simulink model "ee463_project_simulationV4"  (R2023b)
settings: Solver=VariableStepAuto  StartTime=0.0  StopTime=0.04  RelTol=1e-3
undefined symbols (not defined in the file or in its folder): Acid, Lead
libraries: spsDiodeLib x8, spsVoltageMeasurementLib x7, spsMeanLib x6, spsCurrentMeasurementLib x5, spsSeriesRLCBranchLib x5, spsACVoltageSourceLib x3, spsBatteryLib x1, spsMosfetLib x1, spsRMSLib x1, sps_lib x1
settings Model: Creator=Emir  LastModifiedBy=Emir

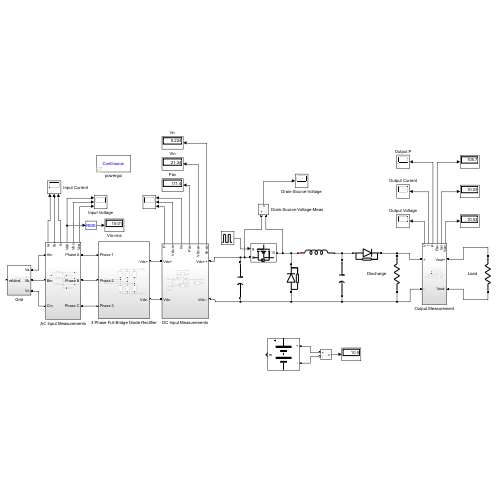
[thumbnail: Simulink's stored preview of the top-level diagram]
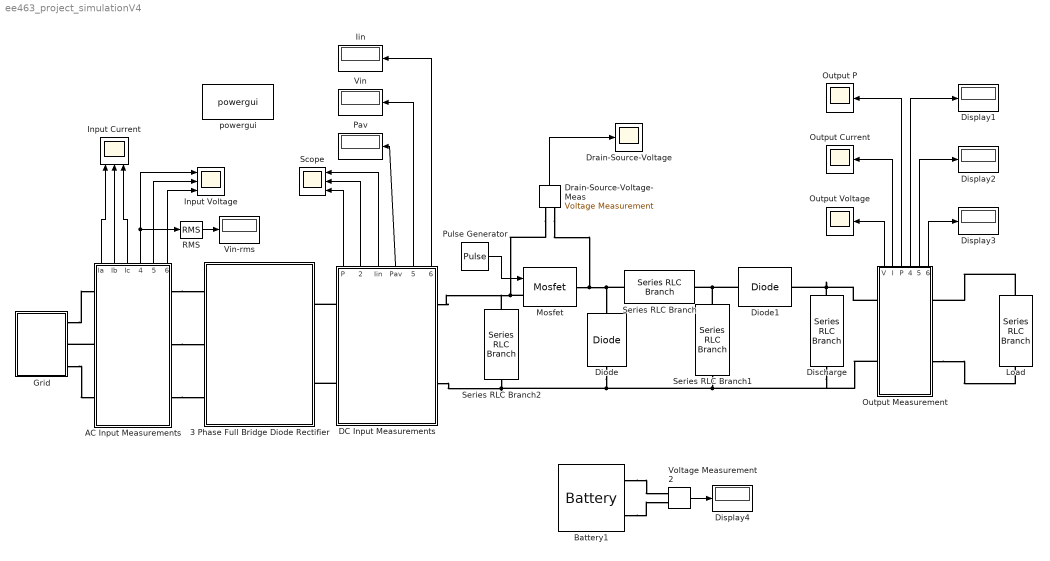
== system ee463_project_simulationV4 ==
  3 Phase Full Bridge Diode Rectifier : Subsystem
  AC Input Measurements : Subsystem
      settings: PortSchema="{\"entries\":[{\"content\":{\"sides\":[{\"content\":{\"connectorIds\":[\"LConn1\",\"LConn2\",\"LConn3\"]},\"type\":\"ConnectorPlacement.EquallySpacedRectSide\",\"uuid\":\"04a5a0c8-76ab-4056-bfdd-b703a3d2aa28\"},{\"content\":{\"connectorIds\":[\"RConn1\",\"RConn2\",\"RConn3\"],\"side\":\"RIGHT\"},\"type\":\"ConnectorPlacement.EquallySpacedRectSide\",\"uuid\":\"3565172a-00f9-43c9-81c3-3e47c8c41d3a\"},{\"content\":{\"connectorIds\":[\"Out1\",\"Out2\",\"Out3\",\"Out4\",\"Out5\",\"Out6\"],\"side\":\"TOP\"},\"type\":\"ConnectorPlacement.EquallySpacedRectSide\",\"uuid\":\"dbadec88-7628-4dba-94e1-272ca81af1aa\"},{\"content\":{\"side\":\"BOTTOM\"},\"type\":\"ConnectorPlacement.EquallySpacedRectSide\",\"uuid\":\"5d01f6b5-6790-4bc6-9328-17bbb75a6f10\"}]},\"type\":\"ConnectorPlacement.EquallySpacedConnector\",\"uuid\":\"addb2cae-2f57-4e8c-a556-dd1f5358b3e0\"}],\"packageUris\":[\"http://schema.mathworks.com/mf0/Connector/R2020b\"],\"version\":\"1.0\"}"
  Battery1 : spsBatteryLib/Battery  BatType=Lead-Acid  ShowTempParam=off  ThermalPreset=no  ShowAgeParam=off  NomV=12  NomQ=100  SOC=10  Batt_Tr=30  PresetModel=on  MaxQ=104.1667  MinV=9  FullV=13.0658  Dis_rate=20  R=0.0012  Normal_OP=31.0278  expZone="[12.2171     0.333333]"  current=[6.5 13 32.5]  Units=Time  Tci=20  NomT=20  T2=-30  MaxQ2=4.8  FullV2=7.1  Normal_OP2=5.655  expZone2="[6.58           1]"  Rca=0.6  ti=2000  Dp=0  Neq0=0  Tsim=1e6  Ta1=25  Qeol=5.4*0.9  Reol=0.013333*1.2  Char_age=[2.3478, 3]  Dis_age=[2.3478, 10]  N1=1500  N2=10500  N3=1000  N4=1400  Ta2=45  N5=950
  DC Input Measurements : Subsystem
      settings: PortSchema="{\"entries\":[{\"content\":{\"sides\":[{\"content\":{\"connectorIds\":[\"LConn1\",\"LConn2\"]},\"type\":\"ConnectorPlacement.EquallySpacedRectSide\",\"uuid\":\"d21f3327-f92a-42ff-962f-d2a0482b5819\"},{\"content\":{\"connectorIds\":[\"RConn1\",\"RConn2\"],\"side\":\"RIGHT\"},\"type\":\"ConnectorPlacement.EquallySpacedRectSide\",\"uuid\":\"4cc980a8-4b33-4409-8260-8c3cf4970e9e\"},{\"content\":{\"connectorIds\":[\"Out1\",\"Out2\",\"Out3\",\"Out4\",\"Out5\",\"Out6\"],\"side\":\"TOP\"},\"type\":\"ConnectorPlacement.EquallySpacedRectSide\",\"uuid\":\"010d1ec9-7ee7-4226-b983-8384f0725a58\"},{\"content\":{\"side\":\"BOTTOM\"},\"type\":\"ConnectorPlacement.EquallySpacedRectSide\",\"uuid\":\"5c959f18-9408-4ec5-8d60-b5cac5d211f5\"}]},\"type\":\"ConnectorPlacement.EquallySpacedConnector\",\"uuid\":\"5b7df6e5-50e0-402e-8feb-d27b87324437\"}],\"packageUris\":[\"http://schema.mathworks.com/mf0/Connector/R2020b\"],\"version\":\"1.0\"}"
  Diode : spsDiodeLib/Diode  Ron=0.001  Lon=0  Vf=0.8  IC=0  UseSnubber=0  Rs=500  Cs=250e-9  Measurements=off
  Diode1 : spsDiodeLib/Diode  Ron=0.001  Lon=0  Vf=0.8  IC=0  UseSnubber=0  Rs=500  Cs=250e-9  Measurements=off
  Discharge : spsSeriesRLCBranchLib/Series RLC Branch  LConnTagsString=__new0  RConnTagsString=__new0  BranchType=R  Resistance=100000  Inductance=1e-3  SetiL0=off  InitialCurrent=0  Capacitance=1000e-6  Setx0=off  InitialVoltage=0  Measurements=None
  Display{1..4} (4 alike) : Display
  Drain-Source-Voltage : Scope
  Drain-Source-Voltage-Meas : spsVoltageMeasurementLib/Voltage Measurement  PhasorSimulation=off  OutputType=Complex  PSBequivalent=0
  Grid : Subsystem
  Iin : Display
  Input Current : Scope  NumInputPorts=3
  Input Voltage : Scope  NumInputPorts=3
  Load : spsSeriesRLCBranchLib/Series RLC Branch  LConnTagsString=__new0  RConnTagsString=__new0  BranchType=R  Resistance=1.05  Inductance=1e-3  SetiL0=off  InitialCurrent=0  Capacitance=1000e-6  Setx0=off  InitialVoltage=0  Measurements=None
  Mosfet : spsMosfetLib/Mosfet  Ron=0.1  Lon=0  Rd=0.01  Vfd=0  IC=0  Rs=1e5  Cs=inf  Measurements=off
  Output Current : Scope
  Output Measurement : Subsystem
      settings: PortSchema="{\"entries\":[{\"content\":{\"sides\":[{\"content\":{\"connectorIds\":[\"LConn1\",\"LConn2\"]},\"type\":\"ConnectorPlacement.EquallySpacedRectSide\",\"uuid\":\"5134c9a7-91fc-4055-8b38-7fcc39efd9ae\"},{\"content\":{\"connectorIds\":[\"RConn1\",\"RConn2\"],\"side\":\"RIGHT\"},\"type\":\"ConnectorPlacement.EquallySpacedRectSide\",\"uuid\":\"a0adcaf9-cd58-4f8e-859e-0ced41501c8a\"},{\"content\":{\"connectorIds\":[\"Out1\",\"Out2\",\"Out3\",\"Out4\",\"Out5\",\"Out6\"],\"side\":\"TOP\"},\"type\":\"ConnectorPlacement.EquallySpacedRectSide\",\"uuid\":\"15bd731c-c78b-43c7-93d7-93e7c2271690\"}]},\"type\":\"ConnectorPlacement.EquallySpacedConnector\",\"uuid\":\"f842e8ba-c63a-4c27-b4ce-14ca0dc73f48\"}],\"packageUris\":[\"http://schema.mathworks.com/mf0/Connector/R2020b\"],\"version\":\"1.0\"}"
  Output P : Scope
  Output Voltage : Scope
  Pav : Display
  Pulse Generator : DiscretePulseGenerator  PulseType=Time based  Period=1e-5  PulseWidth=51.84
  RMS : spsRMSLib/RMS  TrueRMS=on  Freq=60  RMSInit=120  Ts=0
  Scope : Scope  NumInputPorts=3
  Series RLC Branch : spsSeriesRLCBranchLib/Series RLC Branch  LConnTagsString=__new0  RConnTagsString=__new0  BranchType=L  Resistance=1  Inductance=100e-6  SetiL0=off  InitialCurrent=0  Capacitance=1e-6  Setx0=off  InitialVoltage=0  Measurements=None
  Series RLC Branch1 : spsSeriesRLCBranchLib/Series RLC Branch  LConnTagsString=__new0  RConnTagsString=__new0  BranchType=C  Resistance=100  Inductance=1e-3  SetiL0=off  InitialCurrent=0  Capacitance=5.6e-6  Setx0=off  InitialVoltage=0  Measurements=None
  Series RLC Branch2 : spsSeriesRLCBranchLib/Series RLC Branch  LConnTagsString=__new0  RConnTagsString=__new0  BranchType=C  Resistance=100  Inductance=1e-3  SetiL0=off  InitialCurrent=0  Capacitance=4000e-6  Setx0=off  InitialVoltage=0  Measurements=None
  Vin : Display
  Vin-rms : Display
  Voltage Measurement2 : spsVoltageMeasurementLib/Voltage Measurement  PhasorSimulation=off  OutputType=Complex  PSBequivalent=0
  powergui : sps_lib/powergui  Priority=1  SimulationMode=Continuous  SampleTime=50e-6  frequency=60  Iterations=50  frequencyindice=0  Pbase=100e6  ErrMax=1e-4  UnitsV=kV  UnitsW=MW  buscounter=0  FunctionMessages=off  echomessages=off  EnableUseOfTLC=off  CurrentSourceSwitches=off  DisableSnubberDevices=off  DisableRonSwitches=off  DisableVfSwitches=on  DisplayEquations=off  AutomaticDiscreteSolvers=off  SolverType=Tustin/Backward Euler (TBE)  Interpol=off  ExternalGateDelay=off  methode=off  Ts=100  x0status=blocks  SPID=on  SwTol=0  HookPort=off  NonlinearTolerance=1e-4  nMaxIteration=100  ContinueOnMaxIteration=off  RestoreLinks=warning  ResistiveCurrentMeasurement=off  Frange=[0:2:500]  Ylog=off  Xlog=on  ShowGrid=off  save=off  variable=ZData  structure=0  ZoomFFT=off  StartTime=0.0  cycles=1  DisplayStyle=1  fundamental=60  FreqAxis=off  MaxFrequency=1000  frequencyindicesteady=1  RmsSteady=1  display=off
  wires:
  Pulse Generator/1 -> Mosfet/1
  Drain-Source-Voltage-Meas/1 -> Drain-Source-Voltage/1
  AC Input Measurements/1(Ia) -> Input Current/1
  AC Input Measurements/4(Vab) -> Input Voltage/1, RMS/1
  AC Input Measurements/2(Ib) -> Input Current/2
  AC Input Measurements/5(Vbc) -> Input Voltage/2
  AC Input Measurements/3(Ic) -> Input Current/3
  RMS/1 -> Vin-rms/1
  Voltage Measurement2/1 -> Display4/1
  DC Input Measurements/5(Vdc-av) -> Vin/1
  DC Input Measurements/6(Iin-av) -> Iin/1
  DC Input Measurements/1(P) -> Scope/3
  DC Input Measurements/4(Pav) -> Pav/1
  AC Input Measurements/6(Vca) -> Input Voltage/3
  DC Input Measurements/2(Vdc-in) -> Scope/2
  DC Input Measurements/3(Iin) -> Scope/1
  Output Measurement/2(I) -> Output Current/1
  Output Measurement/1(V) -> Output Voltage/1
  Output Measurement/3(P) -> Output P/1
  Output Measurement/6(V-av) -> Display3/1
  Output Measurement/5(Iav) -> Display2/1
  Output Measurement/4(Pav) -> Display1/1
  connections:
  DC Input Measurements/LConn2 -- 3 Phase Full Bridge Diode Rectifier/RConn2
  Drain-Source-Voltage-Meas/LConn1 -- DC Input Measurements/RConn1 -- Series RLC Branch2/LConn1 -- Mosfet/LConn1
  Mosfet/RConn1 -- Series RLC Branch/LConn1 -- Diode/RConn1 -- Drain-Source-Voltage-Meas/LConn2
  Series RLC Branch1/LConn1 -- Diode1/LConn1 -- Series RLC Branch/RConn1
  AC Input Measurements/RConn1 -- 3 Phase Full Bridge Diode Rectifier/LConn1
  Grid/RConn1 -- AC Input Measurements/LConn1
  AC Input Measurements/LConn2 -- Grid/RConn2
  AC Input Measurements/RConn2 -- 3 Phase Full Bridge Diode Rectifier/LConn2
  Grid/RConn3 -- AC Input Measurements/LConn3
  AC Input Measurements/RConn3 -- 3 Phase Full Bridge Diode Rectifier/LConn3
  Battery1/LConn1 -- Voltage Measurement2/LConn1
  Battery1/LConn2 -- Voltage Measurement2/LConn2
  DC Input Measurements/LConn1 -- 3 Phase Full Bridge Diode Rectifier/RConn1
  Series RLC Branch1/RConn1 -- Discharge/RConn1 -- Output Measurement/LConn2 -- DC Input Measurements/RConn2 -- Series RLC Branch2/RConn1 -- Diode/LConn1
  Output Measurement/LConn1 -- Diode1/RConn1 -- Discharge/LConn1
  Load/LConn1 -- Output Measurement/RConn1
  Output Measurement/RConn2 -- Load/RConn1

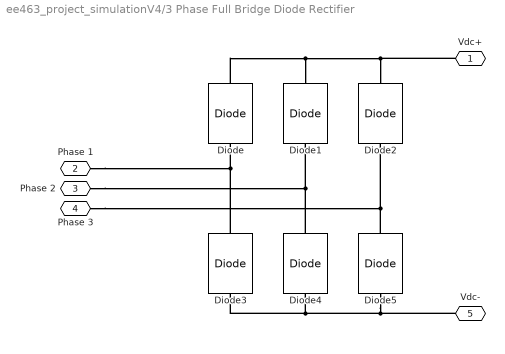
== system ee463_project_simulationV4/3 Phase Full Bridge Diode Rectifier ==
  Diode{,1..5} (6 alike) : spsDiodeLib/Diode  Ron=0.001  Lon=0  Vf=0.8  IC=0  UseSnubber=0  Rs=500  Cs=250e-9  Measurements=off
  Vdc+ : PMIOPort  Side=Right
  Phase 1 : PMIOPort  Port=2  Side=Left
  Phase 2 : PMIOPort  Port=3  Side=Left
  Phase 3 : PMIOPort  Port=4  Side=Left
  Vdc- : PMIOPort  Port=5  Side=Right
  connections:
  Diode4/RConn1 -- Phase 2/RConn1 -- Diode1/LConn1
  Diode5/RConn1 -- Phase 3/RConn1 -- Diode2/LConn1
  Diode/RConn1 -- Diode1/RConn1 -- Vdc+/RConn1 -- Diode2/RConn1
  Diode3/RConn1 -- Phase 1/RConn1 -- Diode/LConn1
  Diode5/LConn1 -- Vdc-/RConn1 -- Diode4/LConn1 -- Diode3/LConn1

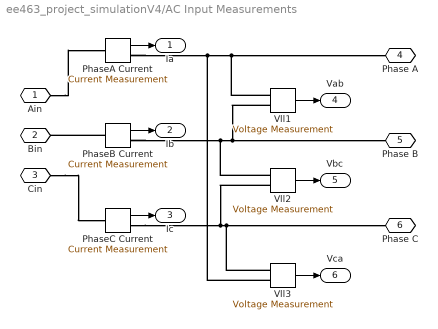
== system ee463_project_simulationV4/AC Input Measurements ==
  PhaseA Current : spsCurrentMeasurementLib/Current Measurement  PhasorSimulation=off  OutputType=Complex  PSBequivalent=0
  PhaseB Current : spsCurrentMeasurementLib/Current Measurement  PhasorSimulation=off  OutputType=Complex  PSBequivalent=0
  PhaseC Current : spsCurrentMeasurementLib/Current Measurement  PhasorSimulation=off  OutputType=Complex  PSBequivalent=0
  Vll1 : spsVoltageMeasurementLib/Voltage Measurement  PhasorSimulation=off  OutputType=Complex  PSBequivalent=0
  Vll2 : spsVoltageMeasurementLib/Voltage Measurement  PhasorSimulation=off  OutputType=Complex  PSBequivalent=0
  Vll3 : spsVoltageMeasurementLib/Voltage Measurement  PhasorSimulation=off  OutputType=Complex  PSBequivalent=0
  Ain : PMIOPort  Side=Left
  Bin : PMIOPort  Port=2  Side=Left
  Cin : PMIOPort  Port=3  Side=Left
  Phase A : PMIOPort  Port=4  Side=Right
  Phase B : PMIOPort  Port=5  Side=Right
  Phase C : PMIOPort  Port=6  Side=Right
  Ia : Outport
  Ib : Outport  Port=2
  Ic : Outport  Port=3
  Vab : Outport  Port=4
  Vbc : Outport  Port=5
  Vca : Outport  Port=6
  wires:
  PhaseC Current/1 -> Ic/1
  Vll3/1 -> Vca/1
  PhaseA Current/1 -> Ia/1
  PhaseB Current/1 -> Ib/1
  Vll1/1 -> Vab/1
  Vll2/1 -> Vbc/1
  connections:
  PhaseB Current/RConn1 -- Vll2/LConn1 -- Vll1/LConn2 -- Phase B/RConn1
  PhaseA Current/RConn1 -- Vll3/LConn2 -- Phase A/RConn1 -- Vll1/LConn1
  Cin/RConn1 -- PhaseC Current/LConn1
  Ain/RConn1 -- PhaseA Current/LConn1
  PhaseC Current/RConn1 -- Phase C/RConn1 -- Vll3/LConn1 -- Vll2/LConn2
  PhaseB Current/LConn1 -- Bin/RConn1

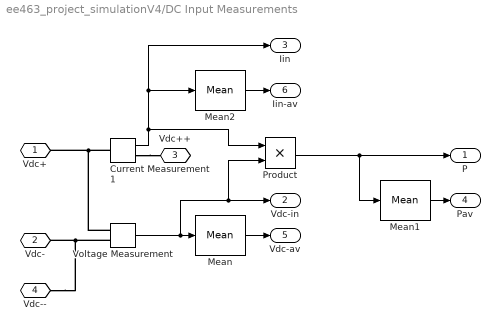
== system ee463_project_simulationV4/DC Input Measurements ==
  Current Measurement1 : spsCurrentMeasurementLib/Current Measurement  PhasorSimulation=off  OutputType=Complex  PSBequivalent=0
  Mean : spsMeanLib/Mean  Freq=60  Vinit=0  Ts=0
  Mean1 : spsMeanLib/Mean  Freq=60  Vinit=0  Ts=0
  Mean2 : spsMeanLib/Mean  Freq=60  Vinit=0  Ts=0
  Product : Product
  Voltage Measurement : spsVoltageMeasurementLib/Voltage Measurement  PhasorSimulation=off  OutputType=Complex  PSBequivalent=0
  Vdc+ : PMIOPort  Side=Left
  Vdc- : PMIOPort  Port=2  Side=Left
  Vdc++ : PMIOPort  Port=3  Side=Right
  Vdc-- : PMIOPort  Port=4  Side=Right
  P : Outport
  Vdc-in : Outport  Port=2
  Iin : Outport  Port=3
  Pav : Outport  Port=4
  Vdc-av : Outport  Port=5
  Iin-av : Outport  Port=6
  wires:
  Current Measurement1/1 -> Iin/1, Mean2/1, Product/1
  Voltage Measurement/1 -> Product/2, Vdc-in/1, Mean/1
  Mean/1 -> Vdc-av/1
  Mean2/1 -> Iin-av/1
  Product/1 -> Mean1/1, P/1
  Mean1/1 -> Pav/1
  connections:
  Current Measurement1/RConn1 -- Vdc++/RConn1
  Current Measurement1/LConn1 -- Voltage Measurement/LConn1 -- Vdc+/RConn1
  Voltage Measurement/LConn2 -- Vdc--/RConn1 -- Vdc-/RConn1

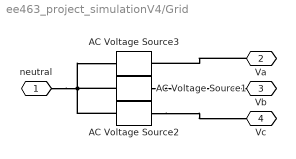
== system ee463_project_simulationV4/Grid ==
  AC Voltage Source1 : spsACVoltageSourceLib/AC Voltage Source  Amplitude=12.8  Phase=-120  Frequency=50  SampleTime=0  Measurements=None  BusType=swing  Pref=10e3  Qref=0  Qmin=-inf  Qmax=+inf
  AC Voltage Source2 : spsACVoltageSourceLib/AC Voltage Source  Amplitude=12.8  Phase=120  Frequency=50  SampleTime=0  Measurements=None  BusType=swing  Pref=10e3  Qref=0  Qmin=-inf  Qmax=+inf
  AC Voltage Source3 : spsACVoltageSourceLib/AC Voltage Source  Amplitude=12.8  Phase=0  Frequency=50  SampleTime=0  Measurements=None  BusType=swing  Pref=10e3  Qref=0  Qmin=-inf  Qmax=+inf
  neutral : PMIOPort  Side=Left
  Va : PMIOPort  Port=2  Side=Right
  Vb : PMIOPort  Port=3  Side=Right
  Vc : PMIOPort  Port=4  Side=Right
  connections:
  AC Voltage Source1/RConn1 -- Vb/RConn1
  Va/RConn1 -- AC Voltage Source3/RConn1
  AC Voltage Source2/RConn1 -- Vc/RConn1
  neutral/RConn1 -- AC Voltage Source3/LConn1 -- AC Voltage Source2/LConn1 -- AC Voltage Source1/LConn1

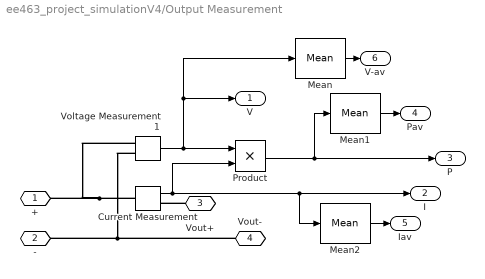
== system ee463_project_simulationV4/Output Measurement ==
  Current Measurement : spsCurrentMeasurementLib/Current Measurement  PhasorSimulation=off  OutputType=Complex  PSBequivalent=0
  Mean : spsMeanLib/Mean  Freq=60  Vinit=0  Ts=0
  Mean1 : spsMeanLib/Mean  Freq=60  Vinit=0  Ts=0
  Mean2 : spsMeanLib/Mean  Freq=60  Vinit=0  Ts=0
  Product : Product
  Voltage Measurement1 : spsVoltageMeasurementLib/Voltage Measurement  PhasorSimulation=off  OutputType=Complex  PSBequivalent=0
  + : PMIOPort  Side=Left
  - : PMIOPort  Port=2  Side=Left
  Vout+ : PMIOPort  Port=3  Side=Right
  Vout- : PMIOPort  Port=4  Side=Right
  V : Outport
  I : Outport  Port=2
  P : Outport  Port=3
  Pav : Outport  Port=4
  Iav : Outport  Port=5
  V-av : Outport  Port=6
  wires:
  Current Measurement/1 -> Mean2/1, I/1, Product/2
  Voltage Measurement1/1 -> Mean/1, V/1, Product/1
  Product/1 -> Mean1/1, P/1
  Mean/1 -> V-av/1
  Mean1/1 -> Pav/1
  Mean2/1 -> Iav/1
  connections:
  Voltage Measurement1/LConn2 -- Vout-/RConn1 -- -/RConn1
  Voltage Measurement1/LConn1 -- +/RConn1 -- Current Measurement/LConn1
  Vout+/RConn1 -- Current Measurement/RConn1
